simulink model "iec_power_meter"  (R2025b)
settings: Solver=VariableStepAuto  StartTime=0.0  StopTime=simlength  RelTol=1e-3
model workspace (MAT data in the model file):
  phi = 0.785398163397
values from neighbouring files (symbols this model uses):
  in_eta_pu = 0.0    (= 0)    [init_model.m]
  in_xi_pu = 0.0    (= 0)    [init_model.m]
  ip_eta_pu = 0.5    [init_model.m]
  ip_xi_pu = 1    [init_model.m]
  ts_afe = 1/fPWM_AFE/2    (= 0.000125)    [init_model.m]
  vn_eta_pu = 0.0    (= 0)    [init_model.m]
  vn_xi_pu = 0.0    (= 0)    [init_model.m]
  vp_xi_pu = 1    [init_model.m]
undefined symbols (not defined in the file or in its folder): I_phase_normalization_factor, omega_grid_emulator_nom, V_phase_normalization_factor
libraries: simple_moving_average_filter x1, simple_moving_average_filter_cc x1, power_meter_iec x1
settings Model: Creator=dbagn  LastModifiedBy=dbagn
settings SFSimCC: SimCustomHeaderCode=|
  | #include "dsmavgflt.h"
  | #include "dsmavgflt_simulink.h"
settings SFSimCC: SimUserSources=|
  | "dsmavgflt_simulink.c"
  | "dsmavgflt.c"
settings SFSimCC: SimUserIncludeDirs=|
  | include
  | src

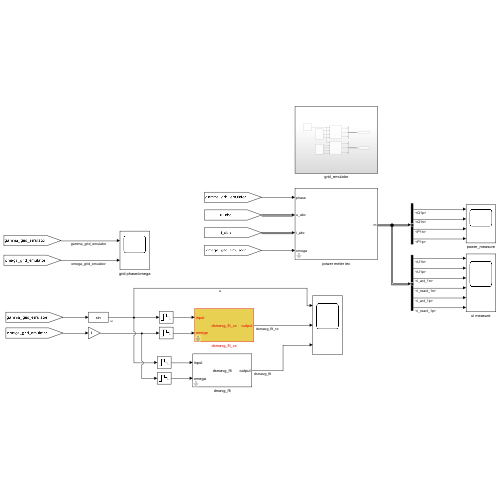
[thumbnail: Simulink's stored preview of the top-level diagram]
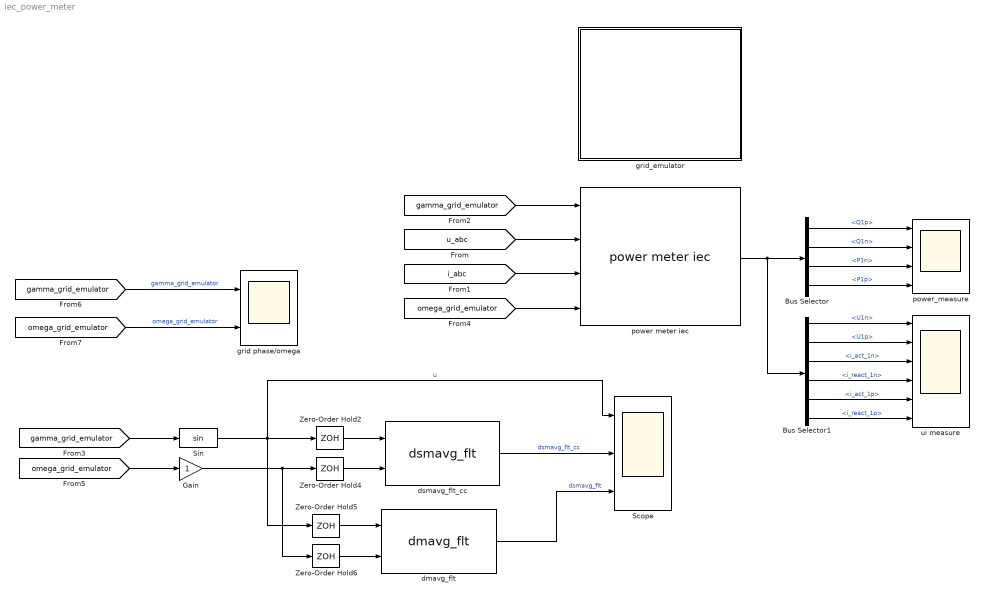
== system iec_power_meter ==
  Bus Selector : BusSelector  OutputSignals=Q1p,Q1n,P1n,P1p
  Bus Selector1 : BusSelector  OutputSignals=U1n,U1p,i_act_1n,i_react_1n,i_act_1p,i_react_1p
  Gain : Gain
  Scope : Scope  NumInputPorts=3
      settings: ActiveDisplayYMinimum=-1.2499998289525023  ActiveDisplayYMaximum=1.2499999809937918  DataLoggingVariableName=ScopeData2
  Sin : Trigonometry
  Zero-Order Hold{2,4..6} (4 alike) : ZeroOrderHold  SampleTime=ts_afe
  dmavg_flt : simple_moving_average_filter/dmavg_flt  ts=ts_afe
  dsmavg_flt_cc : simple_moving_average_filter_cc/dsmavg_flt  instance=0  ts=ts_afe
  grid phase/omega : Scope  NumInputPorts=2
      settings: ActiveDisplayYMinimum=-3.926953707550084  ActiveDisplayYMaximum=3.9269067422486352  DataLoggingVariableName=ScopeData3
  grid_emulator : Subsystem
  power meter iec : power_meter_iec/power meter iec  period=10e-3  ts=ts_afe
  power_measure : Scope  NumInputPorts=4
      settings: ActiveDisplayYMinimum=-181505.02546007198  ActiveDisplayYMaximum=20139.901890231529
  ui measure : Scope  NumInputPorts=6
      settings: ActiveDisplayString=6  ActiveDisplayYMinimum=-151.66666666666714  ActiveDisplayYMaximum=15.00000000000005
  wires:
  [i_abc] -> power meter iec/3
  [u_abc] -> power meter iec/2
  [gamma_grid_emulator] -> power meter iec/1
  power meter iec/1 -> Bus Selector1/1, Bus Selector/1
  Bus Selector/1 -> power_measure/1  "<Q1p>"
  Bus Selector/2 -> power_measure/2  "<Q1n>"
  Bus Selector/3 -> power_measure/3  "<P1n>"
  Bus Selector/4 -> power_measure/4  "<P1p>"
  Bus Selector1/1 -> ui measure/1  "<U1n>"
  Bus Selector1/2 -> ui measure/2  "<U1p>"
  Bus Selector1/3 -> ui measure/3  "<i_act_1n>"
  Bus Selector1/4 -> ui measure/4  "<i_react_1n>"
  Bus Selector1/5 -> ui measure/5  "<i_act_1p>"
  Bus Selector1/6 -> ui measure/6  "<i_react_1p>"
  [gamma_grid_emulator] -> Sin/1
  Zero-Order Hold4/1 -> dsmavg_flt_cc/2
  Zero-Order Hold2/1 -> dsmavg_flt_cc/1
  [omega_grid_emulator] -> power meter iec/4
  Zero-Order Hold5/1 -> dmavg_flt/1
  Zero-Order Hold6/1 -> dmavg_flt/2
  [gamma_grid_emulator] -> grid phase/omega/1  "gamma_grid_emulator"
  [omega_grid_emulator] -> grid phase/omega/2  "omega_grid_emulator"
  [omega_grid_emulator] -> Gain/1
  Sin/1 -> Scope/1, Zero-Order Hold5/1, Zero-Order Hold2/1  "u"
  dsmavg_flt_cc/1 -> Scope/2  "dsmavg_flt_cc"
  dmavg_flt/1 -> Scope/3  "dsmavg_flt"
  Gain/1 -> Zero-Order Hold4/1, Zero-Order Hold6/1

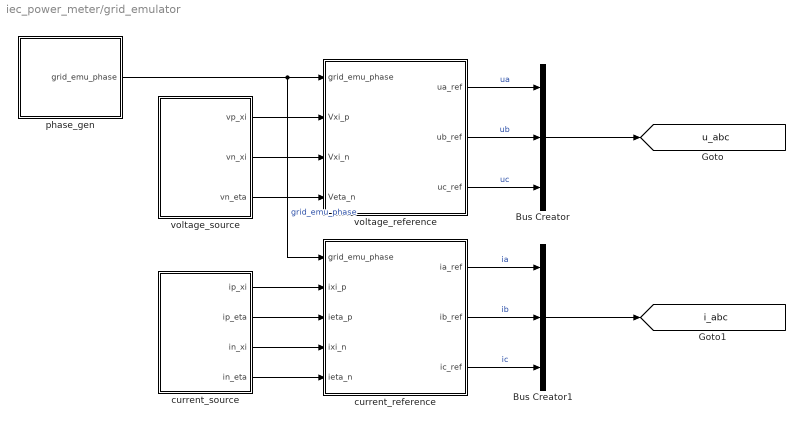
== system iec_power_meter/grid_emulator ==
  Bus Creator : BusCreator  Inputs=3
  Bus Creator1 : BusCreator  Inputs=3
  current_reference : Subsystem
  current_source : Subsystem
  phase_gen : Subsystem
  voltage_reference : Subsystem
  voltage_source : Subsystem
  tag scope: i_abc=global, u_abc=global
  wires:
  phase_gen/1(grid_emu_phase) -> current_reference/1(grid_emu_phase), voltage_reference/1(grid_emu_phase)  "grid_emu_phase"
  voltage_source/2(vn_xi) -> voltage_reference/3(Vxi_n)
  voltage_source/1(vp_xi) -> voltage_reference/2(Vxi_p)
  voltage_source/3(vn_eta) -> voltage_reference/4(Veta_n)
  current_source/4(in_eta) -> current_reference/5(ieta_n)
  current_source/1(ip_xi) -> current_reference/2(ixi_p)
  current_source/3(in_xi) -> current_reference/4(ixi_n)
  current_source/2(ip_eta) -> current_reference/3(ieta_p)
  voltage_reference/2(ub_ref) -> Bus Creator/2  "ub"
  voltage_reference/1(ua_ref) -> Bus Creator/1  "ua"
  voltage_reference/3(uc_ref) -> Bus Creator/3  "uc"
  Bus Creator/1 -> [u_abc]
  Bus Creator1/1 -> [i_abc]
  current_reference/3(ic_ref) -> Bus Creator1/3  "ic"
  current_reference/2(ib_ref) -> Bus Creator1/2  "ib"
  current_reference/1(ia_ref) -> Bus Creator1/1  "ia"

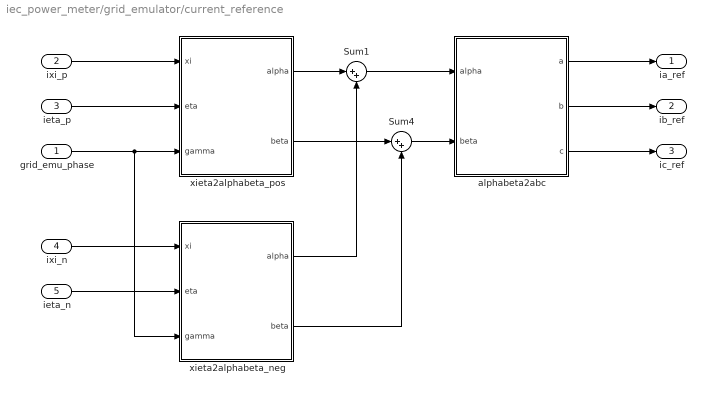
== system iec_power_meter/grid_emulator/current_reference ==
  grid_emu_phase : Inport
  ixi_p : Inport  Port=2
  ieta_p : Inport  Port=3
  ixi_n : Inport  Port=4
  ieta_n : Inport  Port=5
  Sum1 : Sum  Inputs=|++
  Sum4 : Sum  Inputs=|++
  alphabeta2abc : MATLAB Function  TreatAsAtomicUnit=on  SystemSampleTime=ts_afe
  xieta2alphabeta_neg : MATLAB Function  TreatAsAtomicUnit=on  SystemSampleTime=ts_afe
  xieta2alphabeta_pos : MATLAB Function  TreatAsAtomicUnit=on  SystemSampleTime=ts_afe
  ia_ref : Outport  VectorParamsAs1DForOutWhenUnconnected=off
  ib_ref : Outport  Port=2  VectorParamsAs1DForOutWhenUnconnected=off
  ic_ref : Outport  Port=3  VectorParamsAs1DForOutWhenUnconnected=off
  wires:
  ieta_n/1 -> xieta2alphabeta_neg/2(eta)
  ixi_n/1 -> xieta2alphabeta_neg/1(xi)
  ieta_p/1 -> xieta2alphabeta_pos/2(eta)
  ixi_p/1 -> xieta2alphabeta_pos/1(xi)
  grid_emu_phase/1 -> xieta2alphabeta_pos/3(gamma), xieta2alphabeta_neg/3(gamma)
  xieta2alphabeta_neg/2(beta) -> Sum4/2
  xieta2alphabeta_neg/1(alpha) -> Sum1/2
  Sum4/1 -> alphabeta2abc/2(beta)
  xieta2alphabeta_pos/2(beta) -> Sum4/1
  Sum1/1 -> alphabeta2abc/1(alpha)
  xieta2alphabeta_pos/1(alpha) -> Sum1/1
  alphabeta2abc/2(b) -> ib_ref/1
  alphabeta2abc/1(a) -> ia_ref/1
  alphabeta2abc/3(c) -> ic_ref/1

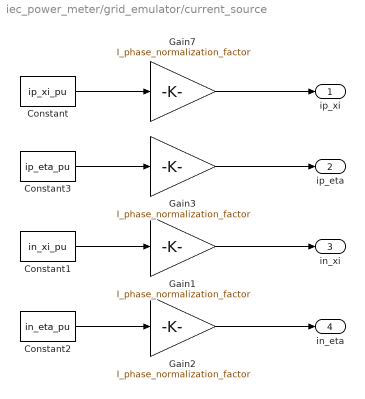
== system iec_power_meter/grid_emulator/current_source ==
  Constant : Constant  Value=ip_xi_pu
  Constant1 : Constant  Value=in_xi_pu
  Constant2 : Constant  Value=in_eta_pu
  Constant3 : Constant  Value=ip_eta_pu
  Gain{1..3,7} (4 alike) : Gain  Gain=I_phase_normalization_factor
  ip_xi : Outport  VectorParamsAs1DForOutWhenUnconnected=off
  ip_eta : Outport  Port=2  VectorParamsAs1DForOutWhenUnconnected=off
  in_xi : Outport  Port=3  VectorParamsAs1DForOutWhenUnconnected=off
  in_eta : Outport  Port=4  VectorParamsAs1DForOutWhenUnconnected=off
  wires:
  Constant2/1 -> Gain2/1
  Constant1/1 -> Gain1/1
  Gain7/1 -> ip_xi/1
  Constant/1 -> Gain7/1
  Gain1/1 -> in_xi/1
  Gain2/1 -> in_eta/1
  Constant3/1 -> Gain3/1
  Gain3/1 -> ip_eta/1

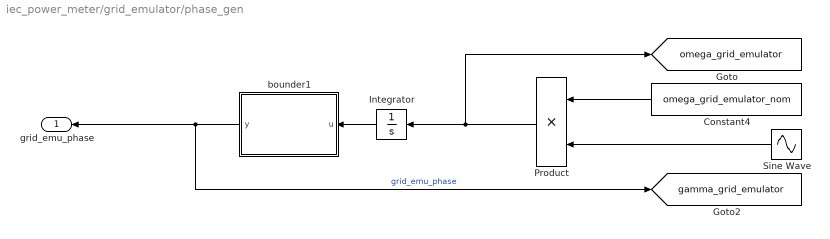
== system iec_power_meter/grid_emulator/phase_gen ==
  Constant4 : Constant  Value=omega_grid_emulator_nom
  Integrator : Integrator
  Product : Product
  Sine Wave : Sin  Amplitude=0  Bias=1  Frequency=2*pi  SampleTime=0
  bounder1 : MATLAB Function  TreatAsAtomicUnit=on  SystemSampleTime=ts_afe
  grid_emu_phase : Outport  VectorParamsAs1DForOutWhenUnconnected=off
  tag scope: gamma_grid_emulator=global, omega_grid_emulator=global
  wires:
  bounder1/1(y) -> [gamma_grid_emulator], grid_emu_phase/1  "grid_emu_phase"
  Integrator/1 -> bounder1/1(u)
  Constant4/1 -> Product/1
  Product/1 -> [omega_grid_emulator], Integrator/1
  Sine Wave/1 -> Product/2

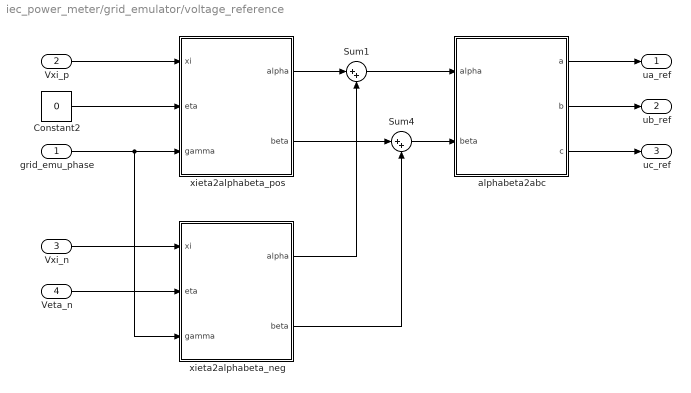
== system iec_power_meter/grid_emulator/voltage_reference ==
  grid_emu_phase : Inport
  Vxi_p : Inport  Port=2
  Vxi_n : Inport  Port=3
  Veta_n : Inport  Port=4
  Constant2 : Constant  Value=0
  Sum1 : Sum  Inputs=|++
  Sum4 : Sum  Inputs=|++
  alphabeta2abc : MATLAB Function  TreatAsAtomicUnit=on  SystemSampleTime=ts_afe
  xieta2alphabeta_neg : MATLAB Function  TreatAsAtomicUnit=on  SystemSampleTime=ts_afe
  xieta2alphabeta_pos : MATLAB Function  TreatAsAtomicUnit=on  SystemSampleTime=ts_afe
  ua_ref : Outport  VectorParamsAs1DForOutWhenUnconnected=off
  ub_ref : Outport  Port=2  VectorParamsAs1DForOutWhenUnconnected=off
  uc_ref : Outport  Port=3  VectorParamsAs1DForOutWhenUnconnected=off
  wires:
  xieta2alphabeta_pos/1(alpha) -> Sum1/1
  Sum1/1 -> alphabeta2abc/1(alpha)
  xieta2alphabeta_pos/2(beta) -> Sum4/1
  Sum4/1 -> alphabeta2abc/2(beta)
  xieta2alphabeta_neg/1(alpha) -> Sum1/2
  xieta2alphabeta_neg/2(beta) -> Sum4/2
  grid_emu_phase/1 -> xieta2alphabeta_neg/3(gamma), xieta2alphabeta_pos/3(gamma)
  Vxi_p/1 -> xieta2alphabeta_pos/1(xi)
  Constant2/1 -> xieta2alphabeta_pos/2(eta)
  Vxi_n/1 -> xieta2alphabeta_neg/1(xi)
  Veta_n/1 -> xieta2alphabeta_neg/2(eta)
  alphabeta2abc/1(a) -> ua_ref/1
  alphabeta2abc/2(b) -> ub_ref/1
  alphabeta2abc/3(c) -> uc_ref/1

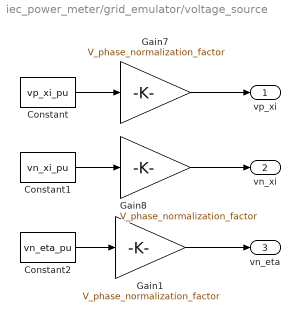
== system iec_power_meter/grid_emulator/voltage_source ==
  Constant : Constant  Value=vp_xi_pu
  Constant1 : Constant  Value=vn_xi_pu
  Constant2 : Constant  Value=vn_eta_pu
  Gain1 : Gain  Gain=V_phase_normalization_factor
  Gain7 : Gain  Gain=V_phase_normalization_factor
  Gain8 : Gain  Gain=V_phase_normalization_factor
  vp_xi : Outport  VectorParamsAs1DForOutWhenUnconnected=off
  vn_xi : Outport  Port=2  VectorParamsAs1DForOutWhenUnconnected=off
  vn_eta : Outport  Port=3  VectorParamsAs1DForOutWhenUnconnected=off
  wires:
  Constant/1 -> Gain7/1
  Constant1/1 -> Gain8/1
  Constant2/1 -> Gain1/1
  Gain7/1 -> vp_xi/1
  Gain8/1 -> vn_xi/1
  Gain1/1 -> vn_eta/1

== matlab function iec_power_meter/grid_emulator/phase_gen/bounder1 ==
  data: u input; y output
function y = bounder(u)    
    y = -pi + mod(u+3*pi,2*pi);
end

== matlab function iec_power_meter/grid_emulator/current_reference/alphabeta2abc ==
  data: alpha input; a output; beta input; b output; c output
function [a,b,c] = alphabeta2abc(alpha,beta)

    a  =  alpha;
    b  =  -0.5*alpha + sqrt(3)/2*beta;
    c  =  -0.5*alpha - sqrt(3)/2*beta;
end

== matlab function iec_power_meter/grid_emulator/voltage_reference/alphabeta2abc ==
  data: alpha input; a output; beta input; b output; c output
function [a,b,c] = alphabeta2abc(alpha,beta)

    a  =  alpha;
    b  =  -0.5*alpha + sqrt(3)/2*beta;
    c  =  -0.5*alpha - sqrt(3)/2*beta;
end

== matlab function iec_power_meter/grid_emulator/voltage_reference/xieta2alphabeta_neg ==
  data: xi input; alpha output; eta input; gamma input; beta output
function [alpha,beta] = xieta2alphabeta_neg(xi,eta,gamma)

    alpha  =  xi*cos(gamma) + eta*sin(gamma);
    beta = -xi*sin(gamma) + eta*cos(gamma);

end

== matlab function iec_power_meter/grid_emulator/current_reference/xieta2alphabeta_neg ==
  data: xi input; alpha output; eta input; gamma input; beta output
function [alpha,beta] = xieta2alphabeta_neg(xi,eta,gamma)

    alpha  =  xi*cos(gamma) + eta*sin(gamma);
    beta = -xi*sin(gamma) + eta*cos(gamma);

end

== matlab function iec_power_meter/grid_emulator/current_reference/xieta2alphabeta_pos ==
  data: xi input; alpha output; eta input; gamma input; beta output
function [alpha,beta] = xieta2alphabeta_pos(xi,eta,gamma)

    alpha  =  xi*cos(gamma) - eta*sin(gamma);
    beta = xi*sin(gamma) + eta*cos(gamma);

end

== matlab function iec_power_meter/grid_emulator/voltage_reference/xieta2alphabeta_pos ==
  data: xi input; alpha output; eta input; gamma input; beta output
function [alpha,beta] = xieta2alphabeta_pos(xi,eta,gamma)

    alpha  =  xi*cos(gamma) - eta*sin(gamma);
    beta = xi*sin(gamma) + eta*cos(gamma);

end
